simulink model "disturbance"  (R2021b)
settings: Solver=VariableStepAuto  StartTime=0.0  StopTime=20  RelTol=1e-3
undefined symbols (not defined in the file or in its folder): den, denG, denG2, num, numG, numG2
settings Model: Creator=ludovicamazzucco  LastModifiedBy=ludovicamazzucco

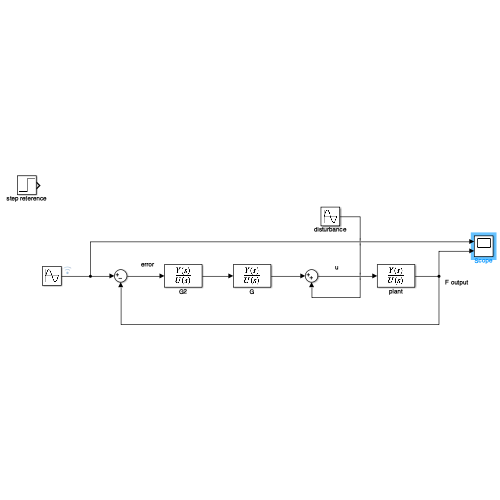
[thumbnail: Simulink's stored preview of the top-level diagram]
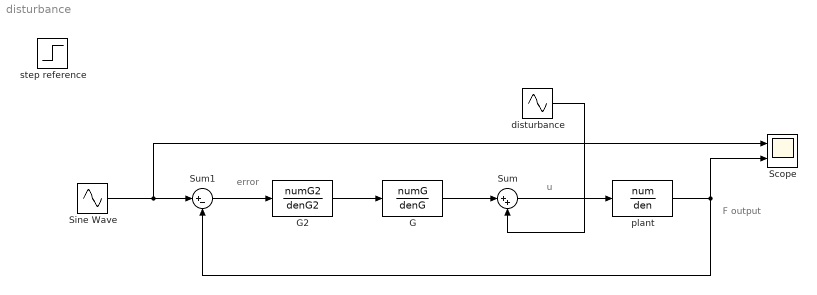
== system disturbance ==
  note: u
  note: F output
  note: error
  G : TransferFcn  Numerator=numG  Denominator=denG
  G2 : TransferFcn  Numerator=numG2  Denominator=denG2
  Scope : Scope  NumInputPorts=2
  Sine Wave : Sin  Frequency=3  SampleTime=0
  Sum : Sum  Inputs=|++
  Sum1 : Sum  Inputs=|+-
  disturbance : Sin  Frequency=3  SampleTime=0
  plant : TransferFcn  Numerator=num  Denominator=den
  step reference : Step  Time=0  SampleTime=0
  wires:
  Sum/1 -> plant/1
  plant/1 -> Scope/2, Sum1/2
  disturbance/1 -> Sum/2
  G2/1 -> G/1
  Sum1/1 -> G2/1
  Sine Wave/1 -> Scope/1, Sum1/1
  G/1 -> Sum/1
